simulink subsystem "controller"  (R2021a)
settings: Solver=VariableStepAuto  StartTime=0.0  StopTime=10.0  RelTol=1e-3
values from neighbouring files (symbols this model uses):
  h10 = par(mode).h10    [quadtank.m]    (also in quadtank_minphase.m = par(1).h10; quadtank_nonminphase.m = par(2).h10; symbolic_linearisation.m = par(2).h10)
  h20 = par(mode).h20    [quadtank.m]    (also in quadtank_minphase.m = par(1).h20; quadtank_nonminphase.m = par(2).h20; symbolic_linearisation.m = par(2).h20)
  K1 = 5    [Task2.m]    (also in Task2_MinimuPhase.m; Task2_Q234mp.m = 6)
  K2 = 5    [Task2.m]    (also in Task2_MinimuPhase.m = 6; Task2_Q234mp.m = 8)
  T1 = 0.5    [Task2.m]    (also in Task2_MinimuPhase.m = 20; Task2_Q234mp.m = 25)
  T2 = 0.5    [Task2.m]    (also in Task2_MinimuPhase.m = 25; Task2_Q234mp.m = 25)
settings Model: Creator=mspms  LastModifiedBy=mspms

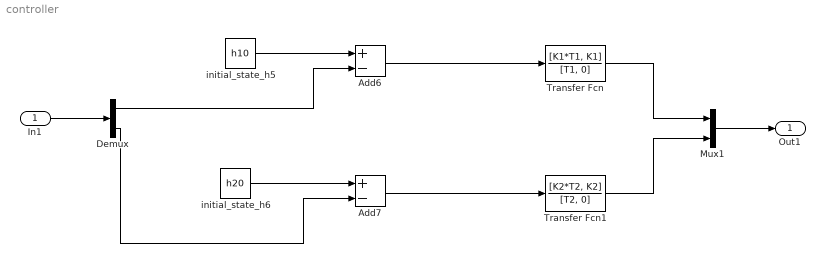
== system controller ==
  In1 : Inport
  Add6 : Sum  Inputs=+-
  Add7 : Sum  Inputs=+-
  Demux : Demux  Outputs=2
  Mux1 : Mux  Inputs=2
  Transfer Fcn : TransferFcn  Numerator=[K1*T1, K1]  Denominator=[T1, 0]
  Transfer Fcn1 : TransferFcn  Numerator=[K2*T2, K2]  Denominator=[T2, 0]
  initial_state_h5 : Constant  Value=h10
  initial_state_h6 : Constant  Value=h20
  Out1 : Outport
  wires:
  Add7/1 -> Transfer Fcn1/1
  Mux1/1 -> Out1/1
  Transfer Fcn1/1 -> Mux1/2
  initial_state_h5/1 -> Add6/1
  Transfer Fcn/1 -> Mux1/1
  Add6/1 -> Transfer Fcn/1
  initial_state_h6/1 -> Add7/1
  In1/1 -> Demux/1
  Demux/1 -> Add6/2
  Demux/2 -> Add7/2
